simulink model "SIL_swarm_Vasarhelyi"  (R2020b)
settings: Solver=FixedStepAuto  StartTime=0.0  StopTime=T  FixedStep=sim_rate  RelTol=1e-3  EnableMultiTasking=on
model workspace (MAT data in the model file):
  SL_ROS_VariableLengthArrays_MaxSizes.CommonInfo.ArrayTruncateAction = 'EmitWarning'
  SL_ROS_VariableLengthArrays_MaxSizes.MsgTypeMap = containers.Map
  SL_ROS_VariableLengthArrays_MaxSizes.MsgTypeMap.serialization.keys = {'aircraft_communication/NetworkComm', 'aircraft_messages/Communication', 'aircraft_messages/NetworkComm'}
  SL_ROS_VariableLengthArrays_MaxSizes.MsgTypeMap.serialization.values{1}.PropertyName = 'Comms'
  SL_ROS_VariableLengthArrays_MaxSizes.MsgTypeMap.serialization.values{1}.DataType = 'aircraft_communication/Communication'
  SL_ROS_VariableLengthArrays_MaxSizes.MsgTypeMap.serialization.values{1}.MaxLength = 4
  SL_ROS_VariableLengthArrays_MaxSizes.MsgTypeMap.serialization.values{2}.PropertyName = 'Ssid'
  SL_ROS_VariableLengthArrays_MaxSizes.MsgTypeMap.serialization.values{2}.DataType = 'uint8'
  SL_ROS_VariableLengthArrays_MaxSizes.MsgTypeMap.serialization.values{2}.MaxLength = 8
  SL_ROS_VariableLengthArrays_MaxSizes.MsgTypeMap.serialization.values{3}.PropertyName = 'Comms'
  SL_ROS_VariableLengthArrays_MaxSizes.MsgTypeMap.serialization.values{3}.DataType = 'aircraft_messages/Communication'
  SL_ROS_VariableLengthArrays_MaxSizes.MsgTypeMap.serialization.values{3}.MaxLength = 8
  SL_ROS_VariableLengthArrays_MaxSizes.MsgTypeMap.serialization.uniformity = 0
  SL_ROS_VariableLengthArrays_MaxSizes.MsgTypeMap.serialization.keyType = 'char'
  SL_ROS_VariableLengthArrays_MaxSizes.MsgTypeMap.serialization.valueType = 'any'
undefined symbols (not defined in the file): airspeed_ref, Altitude_ref, DiscIntNeverNeededParam, Elevators, N_Waypoints, p_swarm, Propeller, Radius_waypoint, RightAileron, RightFlap, Rudder, Waypoints
libraries: robotlib x21, simulink x10, eeGeneralControl x5, dspvision x5
(part 1 of 4)
settings Model: Creator=fcsou  LastModifiedBy=fcsou
settings OptimizationCC: EnhancedBackFolding=on  PassReuseOutputArgsAs=Individual arguments  ZeroExternalMemoryAtStartup=off  ZeroInternalMemoryAtStartup=off  MaxStackSize=64  OptimizeBlockOrder=speed  DifferentSizesBufferReuse=on  OptimizationCustomize=off  EfficientTunableParamExpr=on
settings DebuggingCC: ParameterTunabilityLossMsg=error
settings HardwareCC: ProdBitPerPointer=32  ProdBitPerSizeT=32  ProdBitPerPtrDiffT=32  ProdLargestAtomicFloat=None  ProdIntDivRoundTo=Undefined  ProdEndianess=Unspecified  ProdWordSize=32  ProdHWDeviceType=Generic->Unspecified (assume 32-bit Generic)
settings ModelReferenceCC: PropagateSignalLabelsOutOfModel=off
settings SFSimCC: MATLABDynamicMemAlloc=off
settings RTWCC: Description=Embedded Coder  SystemTargetFile=ert.tlc  HardwareBoard=Robot Operating System (ROS)  TLCOptions="-aInlineSetEventsForThisBaseRateFcn=TLC_FALSE -aSuppressMultiTaskScheduler=TLC_FALSE  -aRateBasedStepFcn=0"  TemplateMakefile=ert_default_tmf  Toolchain=Catkin  TargetLang=C++
settings CodeAppCC: ForceParamTrailComments=on  IgnoreCustomStorageClasses=off  OperatorAnnotations=on  SimulinkDataObjDesc=on  SFDataObjDesc=on  InsertBlockDesc=on
settings ERTTargetCC: ERTCustomFileTemplate=rostime_codertarget_file_process.tlc

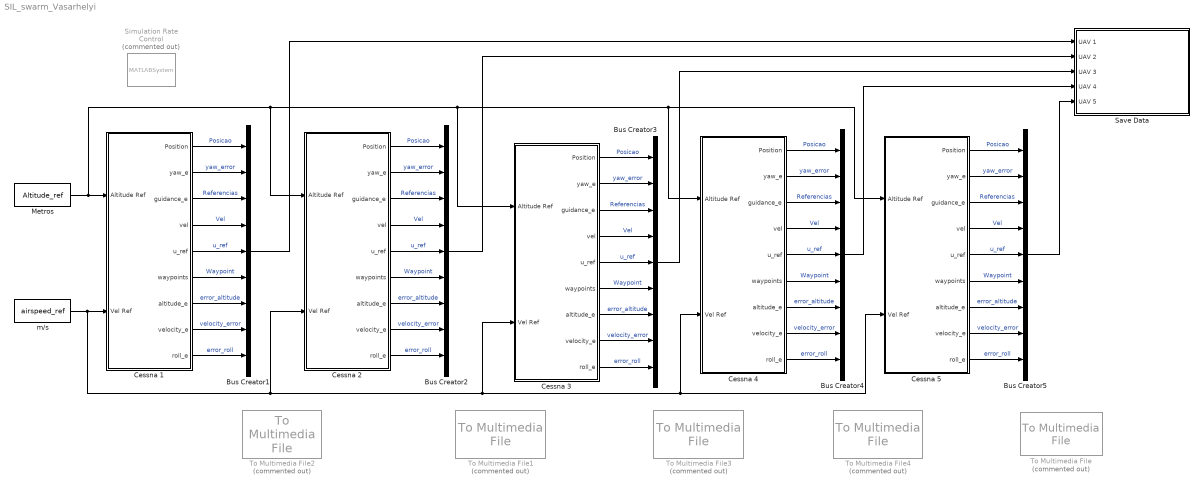
== system SIL_swarm_Vasarhelyi ==
  Bus Creator{1..5} (5 alike) : BusCreator  Inputs=9
  Cessna 1 : Subsystem
  Cessna 2 : Subsystem
  Cessna 3 : Subsystem
  Cessna 4 : Subsystem
  Cessna 5 : Subsystem
  Metros : Constant  Value=Altitude_ref
  Save Data : Subsystem
  Simulation Rate Control : MATLABSystem  Commented=on  System=ExampleHelperSimulationRateControl  SampleTime=0.01
      mask Type: ExampleHelperSimulationRateControl
      mask Display: disp('Rate Control');
  To Multimedia File : dspvision/To Multimedia File  Commented=on  outputFilename=C:\Tese\Results\results_swarm\uav5.mp4  streamSelection=Video only  videoCompressor=Lossy  audioCompressor=None (uncompressed)  imagePorts=One multidimensional signal  fileType=MPEG4  audioDatatype=Determine from input data type  fourcc=RGB  videoQuality=75  mj2000CompFactor=10
  To Multimedia File1 : dspvision/To Multimedia File  Commented=on  outputFilename=C:\Tese\Results\results_swarm\uav2.mp4  streamSelection=Video only  videoCompressor=None (uncompressed)  audioCompressor=None (uncompressed)  imagePorts=One multidimensional signal  fileType=MPEG4  audioDatatype=Determine from input data type  fourcc=RGB  videoQuality=75  mj2000CompFactor=10
  To Multimedia File2 : dspvision/To Multimedia File  Commented=on  outputFilename=C:\Tese\Results\results_swarm\uav1.mp4  streamSelection=Video only  videoCompressor=None (uncompressed)  audioCompressor=None (uncompressed)  imagePorts=One multidimensional signal  fileType=MPEG4  audioDatatype=Determine from input data type  fourcc=RGB  videoQuality=75  mj2000CompFactor=10
  To Multimedia File3 : dspvision/To Multimedia File  Commented=on  outputFilename=C:\Tese\Results\results_swarm\uav3.mp4  streamSelection=Video only  videoCompressor=None (uncompressed)  audioCompressor=None (uncompressed)  imagePorts=One multidimensional signal  fileType=MPEG4  audioDatatype=Determine from input data type  fourcc=RGB  videoQuality=75  mj2000CompFactor=10
  To Multimedia File4 : dspvision/To Multimedia File  Commented=on  outputFilename=C:\Tese\Results\results_swarm\uav4.mp4  streamSelection=Video only  videoCompressor=None (uncompressed)  audioCompressor=None (uncompressed)  imagePorts=One multidimensional signal  fileType=MPEG4  audioDatatype=Determine from input data type  fourcc=RGB  videoQuality=75  mj2000CompFactor=10
  m/s : Constant  Value=airspeed_ref
  wires:
  Bus Creator1/1 -> Save Data/1(UAV 1)
  Cessna 1/4(vel) -> Bus Creator1/4  "Vel"
  Cessna 1/5(u_ref) -> Bus Creator1/5  "u_ref"
  Cessna 1/1(Position) -> Bus Creator1/1  "Posicao"
  Cessna 1/2(yaw_e) -> Bus Creator1/2  "yaw_error"
  Cessna 1/8(velocity_e) -> Bus Creator1/8  "velocity_error"
  Cessna 1/7(altitude_e) -> Bus Creator1/7  "error_altitude"
  Cessna 1/6(waypoints) -> Bus Creator1/6  "Waypoint"
  Cessna 1/3(guidance_e) -> Bus Creator1/3  "Referencias"
  Cessna 1/9(roll_e) -> Bus Creator1/9  "error_roll"
  Cessna 2/9(roll_e) -> Bus Creator2/9  "error_roll"
  Cessna 2/3(guidance_e) -> Bus Creator2/3  "Referencias"
  Cessna 2/8(velocity_e) -> Bus Creator2/8  "velocity_error"
  Cessna 2/7(altitude_e) -> Bus Creator2/7  "error_altitude"
  Cessna 2/4(vel) -> Bus Creator2/4  "Vel"
  Cessna 2/6(waypoints) -> Bus Creator2/6  "Waypoint"
  Cessna 2/1(Position) -> Bus Creator2/1  "Posicao"
  Cessna 2/2(yaw_e) -> Bus Creator2/2  "yaw_error"
  Bus Creator2/1 -> Save Data/2(UAV 2)
  Cessna 2/5(u_ref) -> Bus Creator2/5  "u_ref"
  Cessna 3/9(roll_e) -> Bus Creator3/9  "error_roll"
  Cessna 3/3(guidance_e) -> Bus Creator3/3  "Referencias"
  Cessna 3/8(velocity_e) -> Bus Creator3/8  "velocity_error"
  Cessna 3/7(altitude_e) -> Bus Creator3/7  "error_altitude"
  Cessna 3/4(vel) -> Bus Creator3/4  "Vel"
  Cessna 3/6(waypoints) -> Bus Creator3/6  "Waypoint"
  Cessna 3/1(Position) -> Bus Creator3/1  "Posicao"
  Cessna 3/2(yaw_e) -> Bus Creator3/2  "yaw_error"
  Bus Creator3/1 -> Save Data/3(UAV 3)
  Cessna 3/5(u_ref) -> Bus Creator3/5  "u_ref"
  Cessna 4/9(roll_e) -> Bus Creator4/9  "error_roll"
  Cessna 4/3(guidance_e) -> Bus Creator4/3  "Referencias"
  Cessna 4/8(velocity_e) -> Bus Creator4/8  "velocity_error"
  Cessna 4/7(altitude_e) -> Bus Creator4/7  "error_altitude"
  Cessna 4/4(vel) -> Bus Creator4/4  "Vel"
  Cessna 4/6(waypoints) -> Bus Creator4/6  "Waypoint"
  Cessna 4/1(Position) -> Bus Creator4/1  "Posicao"
  Cessna 4/2(yaw_e) -> Bus Creator4/2  "yaw_error"
  Bus Creator4/1 -> Save Data/4(UAV 4)
  Cessna 4/5(u_ref) -> Bus Creator4/5  "u_ref"
  Metros/1 -> Cessna 4/1(Altitude Ref), Cessna 5/1(Altitude Ref), Cessna 3/1(Altitude Ref), Cessna 2/1(Altitude Ref), Cessna 1/1(Altitude Ref)
  Cessna 5/9(roll_e) -> Bus Creator5/9  "error_roll"
  Cessna 5/3(guidance_e) -> Bus Creator5/3  "Referencias"
  Cessna 5/8(velocity_e) -> Bus Creator5/8  "velocity_error"
  Cessna 5/7(altitude_e) -> Bus Creator5/7  "error_altitude"
  Cessna 5/4(vel) -> Bus Creator5/4  "Vel"
  Cessna 5/6(waypoints) -> Bus Creator5/6  "Waypoint"
  Cessna 5/1(Position) -> Bus Creator5/1  "Posicao"
  m/s/1 -> Cessna 5/2(Vel Ref), Cessna 4/2(Vel Ref), Cessna 3/2(Vel Ref), Cessna 2/2(Vel Ref), Cessna 1/2(Vel Ref)
  Cessna 5/2(yaw_e) -> Bus Creator5/2  "yaw_error"
  Bus Creator5/1 -> Save Data/5(UAV 5)
  Cessna 5/5(u_ref) -> Bus Creator5/5  "u_ref"

== system SIL_swarm_Vasarhelyi/Cessna 1 ==
  Altitude Ref : Inport
  Vel Ref : Inport  Port=2
  Attitude Control : Subsystem
      settings: PortSchema="{\"entries\":[{\"content\":{\"sides\":[{\"content\":{\"connectorIds\":[\"In1\",\"In2\",\"In3\",\"In4\",\"In5\",\"In6\"]},\"type\":\"ConnectorPlacement.EquallySpacedRectSide\",\"uuid\":\"f5987fb5-26bd-460f-ada3-c62a2cc917d9\"},{\"content\":{\"connectorIds\":[\"Out1\",\"Out2\",\"Out3\",\"Out4\"],\"side\":\"RIGHT\"},\"type\":\"ConnectorPlacement.EquallySpacedRectSide\",\"uuid\":\"78b4fbb6-b2d6-45e8-a79e-ccfb1aa742fa\"},{\"content\":{\"connectorIds\":[\"Out5\",\"Out6\",\"Out7\"],\"side\":\"TOP\"},\"type\":\"ConnectorPlacement.EquallySpacedRectSide\",\"uuid\":\"043ac8db-db42-42ba-ba46-d4f45f772f93\"},{\"content\":{\"connectorIds\":[],\"side\":\"HIDDEN\"},\"type\":\"ConnectorPlacement.EquallySpacedRectSide\",\"uuid\":\"557a5d68-6739-4613-818d-4b3751c4f08a\"}]},\"type\":\"ConnectorPlacement.EquallySpacedConnector\",\"uuid\":\"675ce67f-dd1b-4b16-8fb4-2c0be5e81414\"}],\"packageUris\":[\"http://schema.mathworks.com/mf0/Connector/R2020b\"],\"version\":\"1.0\"}"
  Bus Creator : BusCreator  Inputs=3
  Bus Creator1 : BusCreator  Inputs=3
  Bus Selector1 : BusSelector  OutputSignals=X,Y
  Controle de Direção : Subsystem
  High-Level : Subsystem
  ROS Communication : Subsystem
      settings: PortSchema="{\"entries\":[{\"content\":{\"sides\":[{\"content\":{\"connectorIds\":[\"In1\",\"In2\",\"In3\",\"In4\"]},\"type\":\"ConnectorPlacement.EquallySpacedRectSide\",\"uuid\":\"37ffebc2-6d57-4912-9ad0-de0bd75c512d\"},{\"content\":{\"connectorIds\":[\"Out1\",\"Out2\",\"Out3\",\"Out4\",\"Out5\",\"Out6\",\"Out7\"],\"side\":\"RIGHT\"},\"type\":\"ConnectorPlacement.EquallySpacedRectSide\",\"uuid\":\"870d0210-578f-4243-99d2-044c742eeea3\"},{\"content\":{\"connectorIds\":[\"Out8\"],\"side\":\"TOP\"},\"type\":\"ConnectorPlacement.EquallySpacedRectSide\",\"uuid\":\"d294e982-d3b3-4a84-8ae3-ca0953cabd4e\"},{\"content\":{\"connectorIds\":[],\"side\":\"HIDDEN\"},\"type\":\"ConnectorPlacement.EquallySpacedRectSide\",\"uuid\":\"f3838956-1f56-4acd-b9fa-f0f63fa39c9b\"}]},\"type\":\"ConnectorPlacement.EquallySpacedConnector\",\"uuid\":\"f2d40ee8-fbac-425c-83b3-c95127bc648e\"}],\"packageUris\":[\"http://schema.mathworks.com/mf0/Connector/R2020b\"],\"version\":\"1.0\"}"
  Position : Outport
  yaw_e : Outport  Port=2
  guidance_e : Outport  Port=3
  vel : Outport  Port=4
  u_ref : Outport  Port=5
  waypoints : Outport  Port=6
  altitude_e : Outport  Port=7
  velocity_e : Outport  Port=8
  roll_e : Outport  Port=9
  wires:
  Attitude Control/4(Throtlle) -> ROS Communication/4(Throttle)
  ROS Communication/2(Pitch) -> Bus Creator/2  "Pitch"
  Bus Selector1/2 -> Controle de Direção/3(Y)  "<Y>"
  Bus Selector1/1 -> Controle de Direção/2(X)  "<X>"
  Attitude Control/3(Aileron) -> ROS Communication/3(Aileron)
  ROS Communication/8(Xi) -> High-Level/3(Xi)
  Bus Creator/1 -> Attitude Control/2(Euler Angles)
  Attitude Control/2(Rudder) -> ROS Communication/2(Rudder)
  ROS Communication/5(ECEF X) -> Bus Creator1/2  "X"
  Controle de Direção/2(Roll Ref) -> Attitude Control/3(Roll_ref)
  Attitude Control/1(Profundor) -> ROS Communication/1(Profundor)
  Bus Creator1/1 -> Position/1, High-Level/1(Pos), Bus Selector1/1
  ROS Communication/6(ECEF Z) -> Attitude Control/4(Altitude), Bus Creator1/3  "Altitude"
  ROS Communication/7(Velocity) -> Attitude Control/5(Vel_in)
  Altitude Ref/1 -> Attitude Control/6(Altitude ref), High-Level/2(Altitude ref)
  High-Level/1(Y Ref) -> Controle de Direção/4(Y Ref)
  High-Level/2(X Ref) -> Controle de Direção/5(X Ref)
  ROS Communication/3(Yaw) -> Controle de Direção/1(Yaw), Bus Creator/3  "Yaw"
  ROS Communication/4(ECEF Y) -> Bus Creator1/1  "Y"
  ROS Communication/1(Roll) -> Bus Creator/1  "Roll"
  Controle de Direção/1(yaw_error) -> yaw_e/1
  Controle de Direção/3(guidance_error) -> guidance_e/1
  High-Level/3(vel) -> vel/1
  High-Level/4(u_ref) -> u_ref/1
  High-Level/5(Waypoints) -> waypoints/1
  Attitude Control/5(altitude_e) -> altitude_e/1
  Attitude Control/6(velocity_e) -> velocity_e/1
  Vel Ref/1 -> Attitude Control/1(Vel ref)
  Attitude Control/7(roll_e) -> roll_e/1

== system SIL_swarm_Vasarhelyi/Cessna 2 ==
  Altitude Ref : Inport
  Vel Ref : Inport  Port=2
  Attitude Control : Subsystem
      settings: PortSchema="{\"entries\":[{\"content\":{\"sides\":[{\"content\":{\"connectorIds\":[\"In1\",\"In2\",\"In3\",\"In4\",\"In5\",\"In6\"]},\"type\":\"ConnectorPlacement.EquallySpacedRectSide\",\"uuid\":\"f5987fb5-26bd-460f-ada3-c62a2cc917d9\"},{\"content\":{\"connectorIds\":[\"Out1\",\"Out2\",\"Out3\",\"Out4\"],\"side\":\"RIGHT\"},\"type\":\"ConnectorPlacement.EquallySpacedRectSide\",\"uuid\":\"78b4fbb6-b2d6-45e8-a79e-ccfb1aa742fa\"},{\"content\":{\"connectorIds\":[\"Out5\",\"Out6\",\"Out7\"],\"side\":\"TOP\"},\"type\":\"ConnectorPlacement.EquallySpacedRectSide\",\"uuid\":\"043ac8db-db42-42ba-ba46-d4f45f772f93\"},{\"content\":{\"connectorIds\":[],\"side\":\"HIDDEN\"},\"type\":\"ConnectorPlacement.EquallySpacedRectSide\",\"uuid\":\"557a5d68-6739-4613-818d-4b3751c4f08a\"}]},\"type\":\"ConnectorPlacement.EquallySpacedConnector\",\"uuid\":\"675ce67f-dd1b-4b16-8fb4-2c0be5e81414\"}],\"packageUris\":[\"http://schema.mathworks.com/mf0/Connector/R2020b\"],\"version\":\"1.0\"}"
  Bus Creator : BusCreator  Inputs=3
  Bus Creator1 : BusCreator  Inputs=3
  Bus Selector1 : BusSelector  OutputSignals=X,Y
  Controle de Direção : Subsystem
  High-Level : Subsystem
  ROS Communication : Subsystem
      settings: PortSchema="{\"entries\":[{\"content\":{\"sides\":[{\"content\":{\"connectorIds\":[\"In1\",\"In2\",\"In3\",\"In4\"]},\"type\":\"ConnectorPlacement.EquallySpacedRectSide\",\"uuid\":\"37ffebc2-6d57-4912-9ad0-de0bd75c512d\"},{\"content\":{\"connectorIds\":[\"Out1\",\"Out2\",\"Out3\",\"Out4\",\"Out5\",\"Out6\",\"Out7\"],\"side\":\"RIGHT\"},\"type\":\"ConnectorPlacement.EquallySpacedRectSide\",\"uuid\":\"870d0210-578f-4243-99d2-044c742eeea3\"},{\"content\":{\"connectorIds\":[\"Out8\"],\"side\":\"TOP\"},\"type\":\"ConnectorPlacement.EquallySpacedRectSide\",\"uuid\":\"d294e982-d3b3-4a84-8ae3-ca0953cabd4e\"},{\"content\":{\"connectorIds\":[],\"side\":\"HIDDEN\"},\"type\":\"ConnectorPlacement.EquallySpacedRectSide\",\"uuid\":\"f3838956-1f56-4acd-b9fa-f0f63fa39c9b\"}]},\"type\":\"ConnectorPlacement.EquallySpacedConnector\",\"uuid\":\"f2d40ee8-fbac-425c-83b3-c95127bc648e\"}],\"packageUris\":[\"http://schema.mathworks.com/mf0/Connector/R2020b\"],\"version\":\"1.0\"}"
  Position : Outport
  yaw_e : Outport  Port=2
  guidance_e : Outport  Port=3
  vel : Outport  Port=4
  u_ref : Outport  Port=5
  waypoints : Outport  Port=6
  altitude_e : Outport  Port=7
  velocity_e : Outport  Port=8
  roll_e : Outport  Port=9
  wires:
  Attitude Control/4(Throtlle) -> ROS Communication/4(Throttle)
  ROS Communication/2(Pitch) -> Bus Creator/2  "Pitch"
  Bus Selector1/2 -> Controle de Direção/3(Y)  "<Y>"
  Bus Selector1/1 -> Controle de Direção/2(X)  "<X>"
  Attitude Control/3(Aileron) -> ROS Communication/3(Aileron)
  ROS Communication/8(Xi) -> High-Level/3(Xi)
  Bus Creator/1 -> Attitude Control/2(Euler Angles)
  Attitude Control/2(Rudder) -> ROS Communication/2(Rudder)
  ROS Communication/5(ECEF X) -> Bus Creator1/2  "X"
  Controle de Direção/2(Roll Ref) -> Attitude Control/3(Roll_ref)
  Attitude Control/1(Profundor) -> ROS Communication/1(Profundor)
  Bus Creator1/1 -> Position/1, High-Level/1(Pos), Bus Selector1/1
  ROS Communication/6(ECEF Z) -> Attitude Control/4(Altitude), Bus Creator1/3  "Altitude"
  ROS Communication/7(Velocity) -> Attitude Control/5(Vel_in)
  Altitude Ref/1 -> Attitude Control/6(Altitude ref), High-Level/2(Altitude ref)
  High-Level/1(Y Ref) -> Controle de Direção/4(Y Ref)
  High-Level/2(X Ref) -> Controle de Direção/5(X Ref)
  ROS Communication/3(Yaw) -> Controle de Direção/1(Yaw), Bus Creator/3  "Yaw"
  ROS Communication/4(ECEF Y) -> Bus Creator1/1  "Y"
  ROS Communication/1(Roll) -> Bus Creator/1  "Roll"
  Controle de Direção/1(yaw_error) -> yaw_e/1
  Controle de Direção/3(guidance_error) -> guidance_e/1
  High-Level/3(vel) -> vel/1
  High-Level/4(u_ref) -> u_ref/1
  High-Level/5(Waypoints) -> waypoints/1
  Attitude Control/5(altitude_e) -> altitude_e/1
  Attitude Control/6(velocity_e) -> velocity_e/1
  Vel Ref/1 -> Attitude Control/1(Vel ref)
  Attitude Control/7(roll_e) -> roll_e/1

== system SIL_swarm_Vasarhelyi/Cessna 3 ==
  Altitude Ref : Inport
  Vel Ref : Inport  Port=2
  Attitude Control : Subsystem
      settings: PortSchema="{\"entries\":[{\"content\":{\"sides\":[{\"content\":{\"connectorIds\":[\"In1\",\"In2\",\"In3\",\"In4\",\"In5\",\"In6\"]},\"type\":\"ConnectorPlacement.EquallySpacedRectSide\",\"uuid\":\"f5987fb5-26bd-460f-ada3-c62a2cc917d9\"},{\"content\":{\"connectorIds\":[\"Out1\",\"Out2\",\"Out3\",\"Out4\"],\"side\":\"RIGHT\"},\"type\":\"ConnectorPlacement.EquallySpacedRectSide\",\"uuid\":\"78b4fbb6-b2d6-45e8-a79e-ccfb1aa742fa\"},{\"content\":{\"connectorIds\":[\"Out5\",\"Out6\",\"Out7\"],\"side\":\"TOP\"},\"type\":\"ConnectorPlacement.EquallySpacedRectSide\",\"uuid\":\"043ac8db-db42-42ba-ba46-d4f45f772f93\"},{\"content\":{\"connectorIds\":[],\"side\":\"HIDDEN\"},\"type\":\"ConnectorPlacement.EquallySpacedRectSide\",\"uuid\":\"557a5d68-6739-4613-818d-4b3751c4f08a\"}]},\"type\":\"ConnectorPlacement.EquallySpacedConnector\",\"uuid\":\"675ce67f-dd1b-4b16-8fb4-2c0be5e81414\"}],\"packageUris\":[\"http://schema.mathworks.com/mf0/Connector/R2020b\"],\"version\":\"1.0\"}"
  Bus Creator : BusCreator  Inputs=3
  Bus Creator1 : BusCreator  Inputs=3
  Bus Selector1 : BusSelector  OutputSignals=X,Y
  Controle de Direção : Subsystem
  High-Level : Subsystem
  ROS Communication : Subsystem
      settings: PortSchema="{\"entries\":[{\"content\":{\"sides\":[{\"content\":{\"connectorIds\":[\"In1\",\"In2\",\"In3\",\"In4\"]},\"type\":\"ConnectorPlacement.EquallySpacedRectSide\",\"uuid\":\"37ffebc2-6d57-4912-9ad0-de0bd75c512d\"},{\"content\":{\"connectorIds\":[\"Out1\",\"Out2\",\"Out3\",\"Out4\",\"Out5\",\"Out6\",\"Out7\"],\"side\":\"RIGHT\"},\"type\":\"ConnectorPlacement.EquallySpacedRectSide\",\"uuid\":\"870d0210-578f-4243-99d2-044c742eeea3\"},{\"content\":{\"connectorIds\":[\"Out8\"],\"side\":\"TOP\"},\"type\":\"ConnectorPlacement.EquallySpacedRectSide\",\"uuid\":\"d294e982-d3b3-4a84-8ae3-ca0953cabd4e\"},{\"content\":{\"connectorIds\":[],\"side\":\"HIDDEN\"},\"type\":\"ConnectorPlacement.EquallySpacedRectSide\",\"uuid\":\"f3838956-1f56-4acd-b9fa-f0f63fa39c9b\"}]},\"type\":\"ConnectorPlacement.EquallySpacedConnector\",\"uuid\":\"f2d40ee8-fbac-425c-83b3-c95127bc648e\"}],\"packageUris\":[\"http://schema.mathworks.com/mf0/Connector/R2020b\"],\"version\":\"1.0\"}"
  Position : Outport
  yaw_e : Outport  Port=2
  guidance_e : Outport  Port=3
  vel : Outport  Port=4
  u_ref : Outport  Port=5
  waypoints : Outport  Port=6
  altitude_e : Outport  Port=7
  velocity_e : Outport  Port=8
  roll_e : Outport  Port=9
  wires:
  Attitude Control/4(Throtlle) -> ROS Communication/4(Throttle)
  ROS Communication/2(Pitch) -> Bus Creator/2  "Pitch"
  Bus Selector1/2 -> Controle de Direção/3(Y)  "<Y>"
  Bus Selector1/1 -> Controle de Direção/2(X)  "<X>"
  Attitude Control/3(Aileron) -> ROS Communication/3(Aileron)
  ROS Communication/8(Xi) -> High-Level/3(Xi)
  Bus Creator/1 -> Attitude Control/2(Euler Angles)
  Attitude Control/2(Rudder) -> ROS Communication/2(Rudder)
  ROS Communication/5(ECEF X) -> Bus Creator1/2  "X"
  Controle de Direção/2(Roll Ref) -> Attitude Control/3(Roll_ref)
  Attitude Control/1(Profundor) -> ROS Communication/1(Profundor)
  Bus Creator1/1 -> Position/1, High-Level/1(Pos), Bus Selector1/1
  ROS Communication/6(ECEF Z) -> Attitude Control/4(Altitude), Bus Creator1/3  "Altitude"
  ROS Communication/7(Velocity) -> Attitude Control/5(Vel_in)
  Altitude Ref/1 -> Attitude Control/6(Altitude ref), High-Level/2(Altitude ref)
  High-Level/1(Y Ref) -> Controle de Direção/4(Y Ref)
  High-Level/2(X Ref) -> Controle de Direção/5(X Ref)
  ROS Communication/3(Yaw) -> Controle de Direção/1(Yaw), Bus Creator/3  "Yaw"
  ROS Communication/4(ECEF Y) -> Bus Creator1/1  "Y"
  ROS Communication/1(Roll) -> Bus Creator/1  "Roll"
  Controle de Direção/1(yaw_error) -> yaw_e/1
  Controle de Direção/3(guidance_error) -> guidance_e/1
  High-Level/3(vel) -> vel/1
  High-Level/4(u_ref) -> u_ref/1
  High-Level/5(Waypoints) -> waypoints/1
  Attitude Control/5(altitude_e) -> altitude_e/1
  Attitude Control/6(velocity_e) -> velocity_e/1
  Vel Ref/1 -> Attitude Control/1(Vel ref)
  Attitude Control/7(roll_e) -> roll_e/1

== system SIL_swarm_Vasarhelyi/Cessna 4 ==
  Altitude Ref : Inport
  Vel Ref : Inport  Port=2
  Attitude Control : Subsystem
      settings: PortSchema="{\"entries\":[{\"content\":{\"sides\":[{\"content\":{\"connectorIds\":[\"In1\",\"In2\",\"In3\",\"In4\",\"In5\",\"In6\"]},\"type\":\"ConnectorPlacement.EquallySpacedRectSide\",\"uuid\":\"f5987fb5-26bd-460f-ada3-c62a2cc917d9\"},{\"content\":{\"connectorIds\":[\"Out1\",\"Out2\",\"Out3\",\"Out4\"],\"side\":\"RIGHT\"},\"type\":\"ConnectorPlacement.EquallySpacedRectSide\",\"uuid\":\"78b4fbb6-b2d6-45e8-a79e-ccfb1aa742fa\"},{\"content\":{\"connectorIds\":[\"Out5\",\"Out6\",\"Out7\"],\"side\":\"TOP\"},\"type\":\"ConnectorPlacement.EquallySpacedRectSide\",\"uuid\":\"043ac8db-db42-42ba-ba46-d4f45f772f93\"},{\"content\":{\"connectorIds\":[],\"side\":\"HIDDEN\"},\"type\":\"ConnectorPlacement.EquallySpacedRectSide\",\"uuid\":\"557a5d68-6739-4613-818d-4b3751c4f08a\"}]},\"type\":\"ConnectorPlacement.EquallySpacedConnector\",\"uuid\":\"675ce67f-dd1b-4b16-8fb4-2c0be5e81414\"}],\"packageUris\":[\"http://schema.mathworks.com/mf0/Connector/R2020b\"],\"version\":\"1.0\"}"
  Bus Creator : BusCreator  Inputs=3
  Bus Creator1 : BusCreator  Inputs=3
  Bus Selector1 : BusSelector  OutputSignals=X,Y
  Controle de Direção : Subsystem
  High-Level : Subsystem
  ROS Communication : Subsystem
      settings: PortSchema="{\"entries\":[{\"content\":{\"sides\":[{\"content\":{\"connectorIds\":[\"In1\",\"In2\",\"In3\",\"In4\"]},\"type\":\"ConnectorPlacement.EquallySpacedRectSide\",\"uuid\":\"37ffebc2-6d57-4912-9ad0-de0bd75c512d\"},{\"content\":{\"connectorIds\":[\"Out1\",\"Out2\",\"Out3\",\"Out4\",\"Out5\",\"Out6\",\"Out7\"],\"side\":\"RIGHT\"},\"type\":\"ConnectorPlacement.EquallySpacedRectSide\",\"uuid\":\"870d0210-578f-4243-99d2-044c742eeea3\"},{\"content\":{\"connectorIds\":[\"Out8\"],\"side\":\"TOP\"},\"type\":\"ConnectorPlacement.EquallySpacedRectSide\",\"uuid\":\"d294e982-d3b3-4a84-8ae3-ca0953cabd4e\"},{\"content\":{\"connectorIds\":[],\"side\":\"HIDDEN\"},\"type\":\"ConnectorPlacement.EquallySpacedRectSide\",\"uuid\":\"f3838956-1f56-4acd-b9fa-f0f63fa39c9b\"}]},\"type\":\"ConnectorPlacement.EquallySpacedConnector\",\"uuid\":\"f2d40ee8-fbac-425c-83b3-c95127bc648e\"}],\"packageUris\":[\"http://schema.mathworks.com/mf0/Connector/R2020b\"],\"version\":\"1.0\"}"
  Position : Outport
  yaw_e : Outport  Port=2
  guidance_e : Outport  Port=3
  vel : Outport  Port=4
  u_ref : Outport  Port=5
  waypoints : Outport  Port=6
  altitude_e : Outport  Port=7
  velocity_e : Outport  Port=8
  roll_e : Outport  Port=9
  wires:
  Attitude Control/4(Throtlle) -> ROS Communication/4(Throttle)
  ROS Communication/2(Pitch) -> Bus Creator/2  "Pitch"
  Bus Selector1/2 -> Controle de Direção/3(Y)  "<Y>"
  Bus Selector1/1 -> Controle de Direção/2(X)  "<X>"
  Attitude Control/3(Aileron) -> ROS Communication/3(Aileron)
  ROS Communication/8(Xi) -> High-Level/3(Xi)
  Bus Creator/1 -> Attitude Control/2(Euler Angles)
  Attitude Control/2(Rudder) -> ROS Communication/2(Rudder)
  ROS Communication/5(ECEF X) -> Bus Creator1/2  "X"
  Controle de Direção/2(Roll Ref) -> Attitude Control/3(Roll_ref)
  Attitude Control/1(Profundor) -> ROS Communication/1(Profundor)
  Bus Creator1/1 -> Position/1, High-Level/1(Pos), Bus Selector1/1
  ROS Communication/6(ECEF Z) -> Attitude Control/4(Altitude), Bus Creator1/3  "Altitude"
  ROS Communication/7(Velocity) -> Attitude Control/5(Vel_in)
  Altitude Ref/1 -> Attitude Control/6(Altitude ref), High-Level/2(Altitude ref)
  High-Level/1(Y Ref) -> Controle de Direção/4(Y Ref)
  High-Level/2(X Ref) -> Controle de Direção/5(X Ref)
  ROS Communication/3(Yaw) -> Controle de Direção/1(Yaw), Bus Creator/3  "Yaw"
  ROS Communication/4(ECEF Y) -> Bus Creator1/1  "Y"
  ROS Communication/1(Roll) -> Bus Creator/1  "Roll"
  Controle de Direção/1(yaw_error) -> yaw_e/1
  Controle de Direção/3(guidance_error) -> guidance_e/1
  High-Level/3(vel) -> vel/1
  High-Level/4(u_ref) -> u_ref/1
  High-Level/5(Waypoints) -> waypoints/1
  Attitude Control/5(altitude_e) -> altitude_e/1
  Attitude Control/6(velocity_e) -> velocity_e/1
  Vel Ref/1 -> Attitude Control/1(Vel ref)
  Attitude Control/7(roll_e) -> roll_e/1

== system SIL_swarm_Vasarhelyi/Cessna 5 ==
  Altitude Ref : Inport
  Vel Ref : Inport  Port=2
  Attitude Control : Subsystem
      settings: PortSchema="{\"entries\":[{\"content\":{\"sides\":[{\"content\":{\"connectorIds\":[\"In1\",\"In2\",\"In3\",\"In4\",\"In5\",\"In6\"]},\"type\":\"ConnectorPlacement.EquallySpacedRectSide\",\"uuid\":\"f5987fb5-26bd-460f-ada3-c62a2cc917d9\"},{\"content\":{\"connectorIds\":[\"Out1\",\"Out2\",\"Out3\",\"Out4\"],\"side\":\"RIGHT\"},\"type\":\"ConnectorPlacement.EquallySpacedRectSide\",\"uuid\":\"78b4fbb6-b2d6-45e8-a79e-ccfb1aa742fa\"},{\"content\":{\"connectorIds\":[\"Out5\",\"Out6\",\"Out7\"],\"side\":\"TOP\"},\"type\":\"ConnectorPlacement.EquallySpacedRectSide\",\"uuid\":\"043ac8db-db42-42ba-ba46-d4f45f772f93\"},{\"content\":{\"connectorIds\":[],\"side\":\"HIDDEN\"},\"type\":\"ConnectorPlacement.EquallySpacedRectSide\",\"uuid\":\"557a5d68-6739-4613-818d-4b3751c4f08a\"}]},\"type\":\"ConnectorPlacement.EquallySpacedConnector\",\"uuid\":\"675ce67f-dd1b-4b16-8fb4-2c0be5e81414\"}],\"packageUris\":[\"http://schema.mathworks.com/mf0/Connector/R2020b\"],\"version\":\"1.0\"}"
  Bus Creator : BusCreator  Inputs=3
  Bus Creator1 : BusCreator  Inputs=3
  Bus Selector1 : BusSelector  OutputSignals=X,Y
  Controle de Direção : Subsystem
  High-Level : Subsystem
  ROS Communication : Subsystem
      settings: PortSchema="{\"entries\":[{\"content\":{\"sides\":[{\"content\":{\"connectorIds\":[\"In1\",\"In2\",\"In3\",\"In4\"]},\"type\":\"ConnectorPlacement.EquallySpacedRectSide\",\"uuid\":\"37ffebc2-6d57-4912-9ad0-de0bd75c512d\"},{\"content\":{\"connectorIds\":[\"Out1\",\"Out2\",\"Out3\",\"Out4\",\"Out5\",\"Out6\",\"Out7\"],\"side\":\"RIGHT\"},\"type\":\"ConnectorPlacement.EquallySpacedRectSide\",\"uuid\":\"870d0210-578f-4243-99d2-044c742eeea3\"},{\"content\":{\"connectorIds\":[\"Out8\"],\"side\":\"TOP\"},\"type\":\"ConnectorPlacement.EquallySpacedRectSide\",\"uuid\":\"d294e982-d3b3-4a84-8ae3-ca0953cabd4e\"},{\"content\":{\"connectorIds\":[],\"side\":\"HIDDEN\"},\"type\":\"ConnectorPlacement.EquallySpacedRectSide\",\"uuid\":\"f3838956-1f56-4acd-b9fa-f0f63fa39c9b\"}]},\"type\":\"ConnectorPlacement.EquallySpacedConnector\",\"uuid\":\"f2d40ee8-fbac-425c-83b3-c95127bc648e\"}],\"packageUris\":[\"http://schema.mathworks.com/mf0/Connector/R2020b\"],\"version\":\"1.0\"}"
  Position : Outport
  yaw_e : Outport  Port=2
  guidance_e : Outport  Port=3
  vel : Outport  Port=4
  u_ref : Outport  Port=5
  waypoints : Outport  Port=6
  altitude_e : Outport  Port=7
  velocity_e : Outport  Port=8
  roll_e : Outport  Port=9
  wires:
  Attitude Control/4(Throtlle) -> ROS Communication/4(Throttle)
  ROS Communication/2(Pitch) -> Bus Creator/2  "Pitch"
  Bus Selector1/2 -> Controle de Direção/3(Y)  "<Y>"
  Bus Selector1/1 -> Controle de Direção/2(X)  "<X>"
  Attitude Control/3(Aileron) -> ROS Communication/3(Aileron)
  ROS Communication/8(Xi) -> High-Level/3(Xi)
  Bus Creator/1 -> Attitude Control/2(Euler Angles)
  Attitude Control/2(Rudder) -> ROS Communication/2(Rudder)
  ROS Communication/5(ECEF X) -> Bus Creator1/2  "X"
  Controle de Direção/2(Roll Ref) -> Attitude Control/3(Roll_ref)
  Attitude Control/1(Profundor) -> ROS Communication/1(Profundor)
  Bus Creator1/1 -> Position/1, High-Level/1(Pos), Bus Selector1/1
  ROS Communication/6(ECEF Z) -> Attitude Control/4(Altitude), Bus Creator1/3  "Altitude"
  ROS Communication/7(Velocity) -> Attitude Control/5(Vel_in)
  Altitude Ref/1 -> Attitude Control/6(Altitude ref), High-Level/2(Altitude ref)
  High-Level/1(Y Ref) -> Controle de Direção/4(Y Ref)
  High-Level/2(X Ref) -> Controle de Direção/5(X Ref)
  ROS Communication/3(Yaw) -> Controle de Direção/1(Yaw), Bus Creator/3  "Yaw"
  ROS Communication/4(ECEF Y) -> Bus Creator1/1  "Y"
  ROS Communication/1(Roll) -> Bus Creator/1  "Roll"
  Controle de Direção/1(yaw_error) -> yaw_e/1
  Controle de Direção/3(guidance_error) -> guidance_e/1
  High-Level/3(vel) -> vel/1
  High-Level/4(u_ref) -> u_ref/1
  High-Level/5(Waypoints) -> waypoints/1
  Attitude Control/5(altitude_e) -> altitude_e/1
  Attitude Control/6(velocity_e) -> velocity_e/1
  Vel Ref/1 -> Attitude Control/1(Vel ref)
  Attitude Control/7(roll_e) -> roll_e/1

== system SIL_swarm_Vasarhelyi/Save Data ==
  UAV 1 : Inport
  UAV 2 : Inport  Port=2
  UAV 3 : Inport  Port=3
  UAV 4 : Inport  Port=4
  UAV 5 : Inport  Port=5
  Current Time : robotlib/Current Time  OutputFormat=double  SampleTime=-1  ModelName=SIL_swarm_Vasarhelyi
      settings: SourceProductBaseCode=RR
  To Workspace1 : ToWorkspace  VariableName=UAV1  SaveFormat=Timeseries  SampleTime=-1
  To Workspace2 : ToWorkspace  VariableName=UAV2  SaveFormat=Timeseries  SampleTime=-1
  To Workspace3 : ToWorkspace  VariableName=UAV3  SaveFormat=Timeseries  SampleTime=-1
  To Workspace4 : ToWorkspace  VariableName=UAV4  SaveFormat=Timeseries  SampleTime=-1
  To Workspace5 : ToWorkspace  VariableName=UAV5  SaveFormat=Timeseries  SampleTime=-1
  To Workspace6 : ToWorkspace  VariableName=ROStime  SaveFormat=Timeseries  SampleTime=-1
  wires:
  UAV 1/1 -> To Workspace1/1
  UAV 2/1 -> To Workspace2/1
  UAV 3/1 -> To Workspace3/1
  UAV 4/1 -> To Workspace4/1
  UAV 5/1 -> To Workspace5/1
  Current Time/1 -> To Workspace6/1

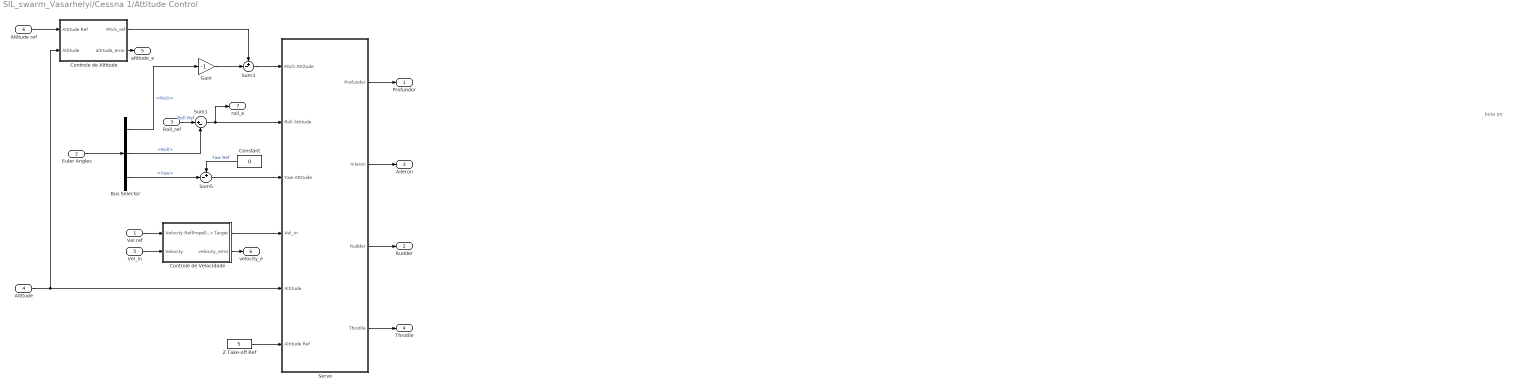
== system SIL_swarm_Vasarhelyi/Cessna 1/Attitude Control ==
  note: bota po
  Vel ref : Inport
  Euler Angles : Inport  Port=2
  Roll_ref : Inport  Port=3
  Altitude : Inport  Port=4
  Vel_in : Inport  Port=5
  Altitude ref : Inport  Port=6
  Bus Selector : BusSelector  OutputSignals=Pitch,Roll,Yaw
  Constant : Constant  Value=0
  Controle de Altitude : Subsystem
  Controle de Velocidade : Subsystem
  Gain : Gain  Gain=-1
  Servo : Subsystem
  Sum1 : Sum  Inputs=|+-
  Sum3 : Sum  Inputs=+-|
  Sum5 : Sum  Inputs=+-|
  Z Take-off Ref : Constant  Value=5
  Profundor : Outport
  Rudder : Outport  Port=2
  Aileron : Outport  Port=3
  Throtlle : Outport  Port=4
  altitude_e : Outport  Port=5
  velocity_e : Outport  Port=6
  roll_e : Outport  Port=7
  wires:
  Roll_ref/1 -> Sum1/1  "Roll Ref"
  Constant/1 -> Sum5/1  "Yaw Ref"
  Servo/4(Throtlle) -> Throtlle/1
  Servo/2(Aileron) -> Aileron/1
  Servo/3(Rudder) -> Rudder/1
  Servo/1(Profundor) -> Profundor/1
  Z Take-off Ref/1 -> Servo/6(Altitude Ref)
  Altitude/1 -> Controle de Altitude/2(Altitude), Servo/5(Altitude)
  Gain/1 -> Sum3/2
  Sum5/1 -> Servo/3(Yaw Attitude)
  Bus Selector/3 -> Sum5/2  "<Yaw>"
  Sum3/1 -> Servo/1(Pitch Attitude)
  Euler Angles/1 -> Bus Selector/1
  Bus Selector/1 -> Gain/1  "<Pitch>"
  Bus Selector/2 -> Sum1/2  "<Roll>"
  Controle de Velocidade/1(Propeller Target) -> Servo/4(Vel_in)
  Controle de Altitude/1(Pitch_ref) -> Sum3/1
  Vel ref/1 -> Controle de Velocidade/1(Velocity Ref)
  Altitude ref/1 -> Controle de Altitude/1(Altitude Ref)
  Sum1/1 -> roll_e/1, Servo/2(Roll Attitude)
  Vel_in/1 -> Controle de Velocidade/2(Velocity)
  Controle de Altitude/2(altitude_error) -> altitude_e/1
  Controle de Velocidade/2(velocity_error) -> velocity_e/1

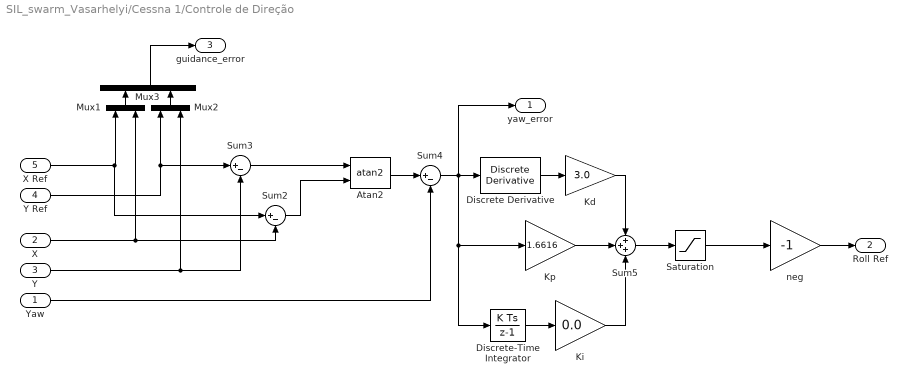
== system SIL_swarm_Vasarhelyi/Cessna 1/Controle de Direção ==
  Yaw : Inport
  X : Inport  Port=2
  Y : Inport  Port=3
  Y Ref : Inport  Port=4
  X Ref : Inport  Port=5
  Atan2 : Trigonometry  Operator=atan2
  Discrete Derivative : simulink/Discrete/Discrete Derivative  gainval=1.0  ICPrevScaledInput=0.0  OutMin=[]  OutMax=[]  OutDataType=fixdt(1, 16)  OutScaling=2^-10  DoSatur=off
  Discrete-Time Integrator : DiscreteIntegrator  SampleTime=-1  ICPrevOutput=DiscIntNeverNeededParam  ICPrevScaledInput=DiscIntNeverNeededParam
  Kd : Gain  Gain=3.0
  Ki : Gain  Gain=0.0
  Kp : Gain  Gain=1.6616
  Mux1 : Mux  Inputs=2
  Mux2 : Mux  Inputs=2
  Mux3 : Mux  Inputs=2
  Saturation : Saturate  UpperLimit=0.226893  LowerLimit=-0.226893
  Sum2 : Sum  Inputs=|+-
  Sum3 : Sum  Inputs=|+-
  Sum4 : Sum  Inputs=|+-
  Sum5 : Sum  Inputs=+++
  neg : Gain  Gain=-1
  yaw_error : Outport
  Roll Ref : Outport  Port=2
  guidance_error : Outport  Port=3
  wires:
  Mux1/1 -> Mux3/1
  Mux2/1 -> Mux3/2
  Saturation/1 -> neg/1
  neg/1 -> Roll Ref/1
  Sum3/1 -> Atan2/1
  Y/1 -> Sum3/2, Mux2/2
  Y Ref/1 -> Sum3/1, Mux2/1
  X Ref/1 -> Sum2/1, Mux1/1
  X/1 -> Sum2/2, Mux1/2
  Sum2/1 -> Atan2/2
  Atan2/1 -> Sum4/1
  Yaw/1 -> Sum4/2
  Mux3/1 -> guidance_error/1
  Sum5/1 -> Saturation/1
  Kp/1 -> Sum5/2
  Kd/1 -> Sum5/1
  Discrete Derivative/1 -> Kd/1
  Discrete-Time Integrator/1 -> Ki/1
  Sum4/1 -> Discrete-Time Integrator/1, Kp/1, Discrete Derivative/1, yaw_error/1
  Ki/1 -> Sum5/3

== system SIL_swarm_Vasarhelyi/Cessna 1/High-Level ==
  Pos : Inport
  Altitude ref : Inport  Port=2
  Xi : Inport  Port=3
  Bus Selector2 : BusSelector  OutputSignals=X,Y,Altitude
  Filtered Derivative Discrete : eeGeneralControl/Filtered Derivative (Discrete or Continuous)  K=1  T=0.001  B=inf  A=-inf  minRatio=10  init_option=Inherited from block input  x0=0  Ts=-1
      settings: SourceProductBaseCode=PS
  Gerador de Waypoints : Subsystem
  Mux : Mux  Inputs=3
  Mux1 : Mux  Inputs=3
  Terminator2 : Terminator
  Vasarhelyi Algorithm : Subsystem
  Velocity Direction : MATLAB Function  TreatAsAtomicUnit=on
  Y Ref : Outport
  X Ref : Outport  Port=2
  vel : Outport  Port=3
  u_ref : Outport  Port=4
  Waypoints : Outport  Port=5
  wires:
  Mux1/1 -> Waypoints/1, Velocity Direction/2(wp)
  Velocity Direction/1(u_ref) -> u_ref/1, Vasarhelyi Algorithm/3(u_ref)
  Pos/1 -> Bus Selector2/1
  Altitude ref/1 -> Mux1/3
  Gerador de Waypoints/2(Y Ref) -> Mux1/2
  Gerador de Waypoints/1(X Ref) -> Mux1/1
  Bus Selector2/1 -> Mux/1  "<X>"
  Bus Selector2/2 -> Mux/2  "<Y>"
  Bus Selector2/3 -> Mux/3  "<Altitude>"
  Mux/1 -> Filtered Derivative Discrete/1, Vasarhelyi Algorithm/1(pos_i), Velocity Direction/1(pos)
  Filtered Derivative Discrete/1 -> vel/1
  Xi/1 -> Vasarhelyi Algorithm/2(pqj)
  Vasarhelyi Algorithm/1(X) -> X Ref/1
  Vasarhelyi Algorithm/2(Y) -> Y Ref/1
  Vasarhelyi Algorithm/3(Z) -> Terminator2/1
  Vasarhelyi Algorithm/4(Xi) -> Gerador de Waypoints/1(Xi)

== system SIL_swarm_Vasarhelyi/Cessna 1/ROS Communication ==
  Profundor : Inport
  Rudder : Inport  Port=2
  Aileron : Inport  Port=3
  Throttle : Inport  Port=4
  Constant : Constant  Value=0
  Constant1 : Constant  Value=0
  Envio e Recepção de Dados do ROS : Subsystem
  Terminator2 : Terminator
  Roll : Outport
  Pitch : Outport  Port=2
  Yaw : Outport  Port=3
  ECEF Y : Outport  Port=4
  ECEF X : Outport  Port=5
  ECEF Z : Outport  Port=6
  Velocity : Outport  Port=7
  Xi : Outport  Port=8
  wires:
  Profundor/1 -> Envio e Recepção de Dados do ROS/2(Elevators)
  Constant/1 -> Envio e Recepção de Dados do ROS/3(Flap)
  Aileron/1 -> Envio e Recepção de Dados do ROS/4(Aileron)
  Envio e Recepção de Dados do ROS/1(Pitch) -> Pitch/1
  Envio e Recepção de Dados do ROS/4(ECEF X) -> ECEF X/1
  Envio e Recepção de Dados do ROS/5(ECEF Y) -> ECEF Y/1
  Envio e Recepção de Dados do ROS/2(Yaw) -> Yaw/1
  Envio e Recepção de Dados do ROS/3(Roll) -> Roll/1
  Envio e Recepção de Dados do ROS/6(ECEF Z) -> ECEF Z/1
  Envio e Recepção de Dados do ROS/7(Velocity) -> Velocity/1
  Rudder/1 -> Terminator2/1
  Envio e Recepção de Dados do ROS/8(Xi) -> Xi/1
  Throttle/1 -> Envio e Recepção de Dados do ROS/5(Propeller)
  Constant1/1 -> Envio e Recepção de Dados do ROS/1(Rudder)

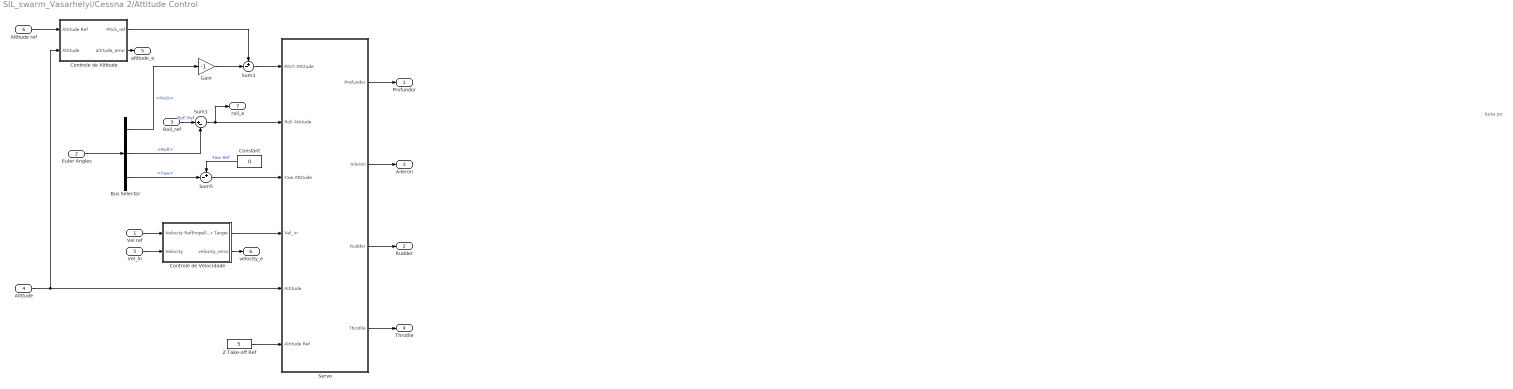
== system SIL_swarm_Vasarhelyi/Cessna 2/Attitude Control ==
  note: bota po
  Vel ref : Inport
  Euler Angles : Inport  Port=2
  Roll_ref : Inport  Port=3
  Altitude : Inport  Port=4
  Vel_in : Inport  Port=5
  Altitude ref : Inport  Port=6
  Bus Selector : BusSelector  OutputSignals=Pitch,Roll,Yaw
  Constant : Constant  Value=0
  Controle de Altitude : Subsystem
  Controle de Velocidade : Subsystem
  Gain : Gain  Gain=-1
  Servo : Subsystem
  Sum1 : Sum  Inputs=|+-
  Sum3 : Sum  Inputs=+-|
  Sum5 : Sum  Inputs=+-|
  Z Take-off Ref : Constant  Value=5
  Profundor : Outport
  Rudder : Outport  Port=2
  Aileron : Outport  Port=3
  Throtlle : Outport  Port=4
  altitude_e : Outport  Port=5
  velocity_e : Outport  Port=6
  roll_e : Outport  Port=7
  wires:
  Roll_ref/1 -> Sum1/1  "Roll Ref"
  Constant/1 -> Sum5/1  "Yaw Ref"
  Servo/4(Throtlle) -> Throtlle/1
  Servo/2(Aileron) -> Aileron/1
  Servo/3(Rudder) -> Rudder/1
  Servo/1(Profundor) -> Profundor/1
  Z Take-off Ref/1 -> Servo/6(Altitude Ref)
  Altitude/1 -> Controle de Altitude/2(Altitude), Servo/5(Altitude)
  Gain/1 -> Sum3/2
  Sum5/1 -> Servo/3(Yaw Attitude)
  Bus Selector/3 -> Sum5/2  "<Yaw>"
  Sum3/1 -> Servo/1(Pitch Attitude)
  Euler Angles/1 -> Bus Selector/1
  Bus Selector/1 -> Gain/1  "<Pitch>"
  Bus Selector/2 -> Sum1/2  "<Roll>"
  Controle de Velocidade/1(Propeller Target) -> Servo/4(Vel_in)
  Controle de Altitude/1(Pitch_ref) -> Sum3/1
  Vel ref/1 -> Controle de Velocidade/1(Velocity Ref)
  Altitude ref/1 -> Controle de Altitude/1(Altitude Ref)
  Sum1/1 -> roll_e/1, Servo/2(Roll Attitude)
  Vel_in/1 -> Controle de Velocidade/2(Velocity)
  Controle de Altitude/2(altitude_error) -> altitude_e/1
  Controle de Velocidade/2(velocity_error) -> velocity_e/1

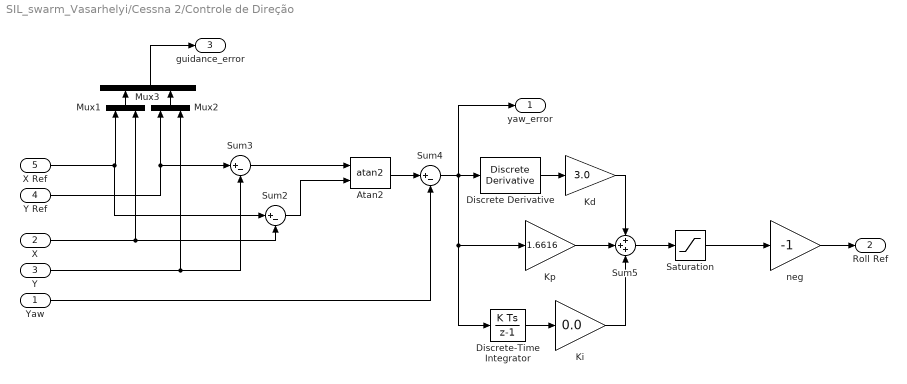
== system SIL_swarm_Vasarhelyi/Cessna 2/Controle de Direção ==
  Yaw : Inport
  X : Inport  Port=2
  Y : Inport  Port=3
  Y Ref : Inport  Port=4
  X Ref : Inport  Port=5
  Atan2 : Trigonometry  Operator=atan2
  Discrete Derivative : simulink/Discrete/Discrete Derivative  gainval=1.0  ICPrevScaledInput=0.0  OutMin=[]  OutMax=[]  OutDataType=fixdt(1, 16)  OutScaling=2^-10  DoSatur=off
  Discrete-Time Integrator : DiscreteIntegrator  SampleTime=-1  ICPrevOutput=DiscIntNeverNeededParam  ICPrevScaledInput=DiscIntNeverNeededParam
  Kd : Gain  Gain=3.0
  Ki : Gain  Gain=0.0
  Kp : Gain  Gain=1.6616
  Mux1 : Mux  Inputs=2
  Mux2 : Mux  Inputs=2
  Mux3 : Mux  Inputs=2
  Saturation : Saturate  UpperLimit=0.226893  LowerLimit=-0.226893
  Sum2 : Sum  Inputs=|+-
  Sum3 : Sum  Inputs=|+-
  Sum4 : Sum  Inputs=|+-
  Sum5 : Sum  Inputs=+++
  neg : Gain  Gain=-1
  yaw_error : Outport
  Roll Ref : Outport  Port=2
  guidance_error : Outport  Port=3
  wires:
  Mux1/1 -> Mux3/1
  Mux2/1 -> Mux3/2
  Saturation/1 -> neg/1
  neg/1 -> Roll Ref/1
  Sum3/1 -> Atan2/1
  Y/1 -> Sum3/2, Mux2/2
  Y Ref/1 -> Sum3/1, Mux2/1
  X Ref/1 -> Sum2/1, Mux1/1
  X/1 -> Sum2/2, Mux1/2
  Sum2/1 -> Atan2/2
  Atan2/1 -> Sum4/1
  Yaw/1 -> Sum4/2
  Mux3/1 -> guidance_error/1
  Sum5/1 -> Saturation/1
  Kp/1 -> Sum5/2
  Kd/1 -> Sum5/1
  Discrete Derivative/1 -> Kd/1
  Discrete-Time Integrator/1 -> Ki/1
  Sum4/1 -> Discrete-Time Integrator/1, Kp/1, Discrete Derivative/1, yaw_error/1
  Ki/1 -> Sum5/3

== system SIL_swarm_Vasarhelyi/Cessna 2/High-Level ==
  Pos : Inport
  Altitude ref : Inport  Port=2
  Xi : Inport  Port=3
  Bus Selector2 : BusSelector  OutputSignals=X,Y,Altitude
  Filtered Derivative Discrete : eeGeneralControl/Filtered Derivative (Discrete or Continuous)  K=1  T=0.001  B=inf  A=-inf  minRatio=10  init_option=Inherited from block input  x0=0  Ts=-1
      settings: SourceProductBaseCode=PS
  Gerador de Waypoints : Subsystem
  Mux : Mux  Inputs=3
  Mux1 : Mux  Inputs=3
  Terminator2 : Terminator
  Vasarhelyi Algorithm : Subsystem
  Velocity Direction : MATLAB Function  TreatAsAtomicUnit=on
  Y Ref : Outport
  X Ref : Outport  Port=2
  vel : Outport  Port=3
  u_ref : Outport  Port=4
  Waypoints : Outport  Port=5
  wires:
  Mux1/1 -> Waypoints/1, Velocity Direction/2(wp)
  Velocity Direction/1(u_ref) -> u_ref/1, Vasarhelyi Algorithm/3(u_ref)
  Pos/1 -> Bus Selector2/1
  Altitude ref/1 -> Mux1/3
  Gerador de Waypoints/2(Y Ref) -> Mux1/2
  Gerador de Waypoints/1(X Ref) -> Mux1/1
  Bus Selector2/1 -> Mux/1  "<X>"
  Bus Selector2/2 -> Mux/2  "<Y>"
  Bus Selector2/3 -> Mux/3  "<Altitude>"
  Mux/1 -> Filtered Derivative Discrete/1, Vasarhelyi Algorithm/1(pos_i), Velocity Direction/1(pos)
  Filtered Derivative Discrete/1 -> vel/1
  Xi/1 -> Vasarhelyi Algorithm/2(pqj)
  Vasarhelyi Algorithm/1(X) -> X Ref/1
  Vasarhelyi Algorithm/2(Y) -> Y Ref/1
  Vasarhelyi Algorithm/3(Z) -> Terminator2/1
  Vasarhelyi Algorithm/4(Xi) -> Gerador de Waypoints/1(Xi)

== system SIL_swarm_Vasarhelyi/Cessna 2/ROS Communication ==
  Profundor : Inport
  Rudder : Inport  Port=2
  Aileron : Inport  Port=3
  Throttle : Inport  Port=4
  Constant : Constant  Value=0
  Constant1 : Constant  Value=0
  Envio e Recepção de Dados do ROS : Subsystem
  Terminator2 : Terminator
  Roll : Outport
  Pitch : Outport  Port=2
  Yaw : Outport  Port=3
  ECEF Y : Outport  Port=4
  ECEF X : Outport  Port=5
  ECEF Z : Outport  Port=6
  Velocity : Outport  Port=7
  Xi : Outport  Port=8
  wires:
  Profundor/1 -> Envio e Recepção de Dados do ROS/2(Elevators)
  Constant/1 -> Envio e Recepção de Dados do ROS/3(Flap)
  Aileron/1 -> Envio e Recepção de Dados do ROS/4(Aileron)
  Envio e Recepção de Dados do ROS/1(Pitch) -> Pitch/1
  Envio e Recepção de Dados do ROS/4(ECEF X) -> ECEF X/1
  Envio e Recepção de Dados do ROS/5(ECEF Y) -> ECEF Y/1
  Envio e Recepção de Dados do ROS/2(Yaw) -> Yaw/1
  Envio e Recepção de Dados do ROS/3(Roll) -> Roll/1
  Envio e Recepção de Dados do ROS/6(ECEF Z) -> ECEF Z/1
  Envio e Recepção de Dados do ROS/7(Velocity) -> Velocity/1
  Rudder/1 -> Terminator2/1
  Envio e Recepção de Dados do ROS/8(Xi) -> Xi/1
  Throttle/1 -> Envio e Recepção de Dados do ROS/5(Propeller)
  Constant1/1 -> Envio e Recepção de Dados do ROS/1(Rudder)

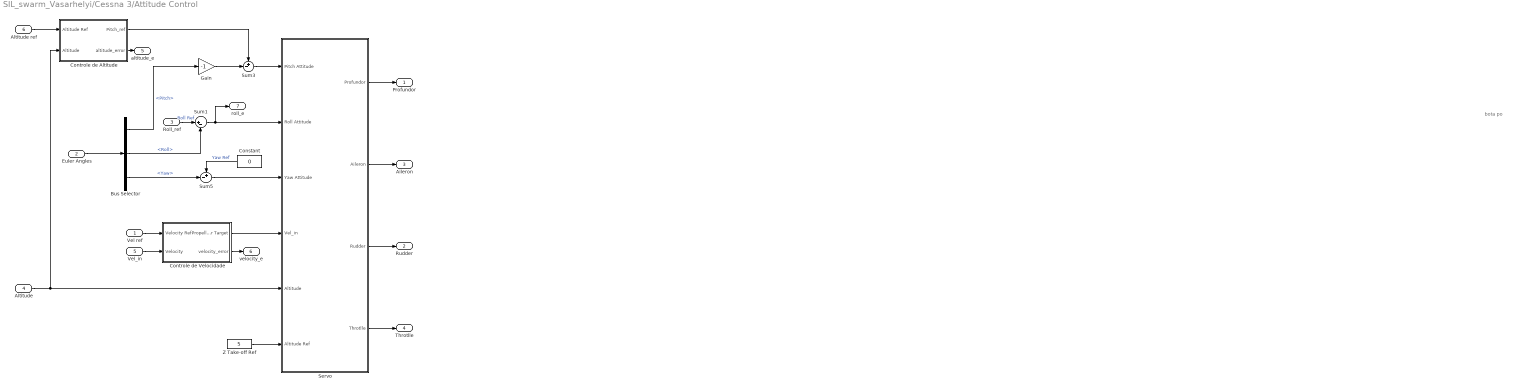
== system SIL_swarm_Vasarhelyi/Cessna 3/Attitude Control ==
  note: bota po
  Vel ref : Inport
  Euler Angles : Inport  Port=2
  Roll_ref : Inport  Port=3
  Altitude : Inport  Port=4
  Vel_in : Inport  Port=5
  Altitude ref : Inport  Port=6
  Bus Selector : BusSelector  OutputSignals=Pitch,Roll,Yaw
  Constant : Constant  Value=0
  Controle de Altitude : Subsystem
  Controle de Velocidade : Subsystem
  Gain : Gain  Gain=-1
  Servo : Subsystem
  Sum1 : Sum  Inputs=|+-
  Sum3 : Sum  Inputs=+-|
  Sum5 : Sum  Inputs=+-|
  Z Take-off Ref : Constant  Value=5
  Profundor : Outport
  Rudder : Outport  Port=2
  Aileron : Outport  Port=3
  Throtlle : Outport  Port=4
  altitude_e : Outport  Port=5
  velocity_e : Outport  Port=6
  roll_e : Outport  Port=7
  wires:
  Roll_ref/1 -> Sum1/1  "Roll Ref"
  Constant/1 -> Sum5/1  "Yaw Ref"
  Servo/4(Throtlle) -> Throtlle/1
  Servo/2(Aileron) -> Aileron/1
  Servo/3(Rudder) -> Rudder/1
  Servo/1(Profundor) -> Profundor/1
  Z Take-off Ref/1 -> Servo/6(Altitude Ref)
  Altitude/1 -> Controle de Altitude/2(Altitude), Servo/5(Altitude)
  Gain/1 -> Sum3/2
  Sum5/1 -> Servo/3(Yaw Attitude)
  Bus Selector/3 -> Sum5/2  "<Yaw>"
  Sum3/1 -> Servo/1(Pitch Attitude)
  Euler Angles/1 -> Bus Selector/1
  Bus Selector/1 -> Gain/1  "<Pitch>"
  Bus Selector/2 -> Sum1/2  "<Roll>"
  Controle de Velocidade/1(Propeller Target) -> Servo/4(Vel_in)
  Controle de Altitude/1(Pitch_ref) -> Sum3/1
  Vel ref/1 -> Controle de Velocidade/1(Velocity Ref)
  Altitude ref/1 -> Controle de Altitude/1(Altitude Ref)
  Sum1/1 -> roll_e/1, Servo/2(Roll Attitude)
  Vel_in/1 -> Controle de Velocidade/2(Velocity)
  Controle de Altitude/2(altitude_error) -> altitude_e/1
  Controle de Velocidade/2(velocity_error) -> velocity_e/1

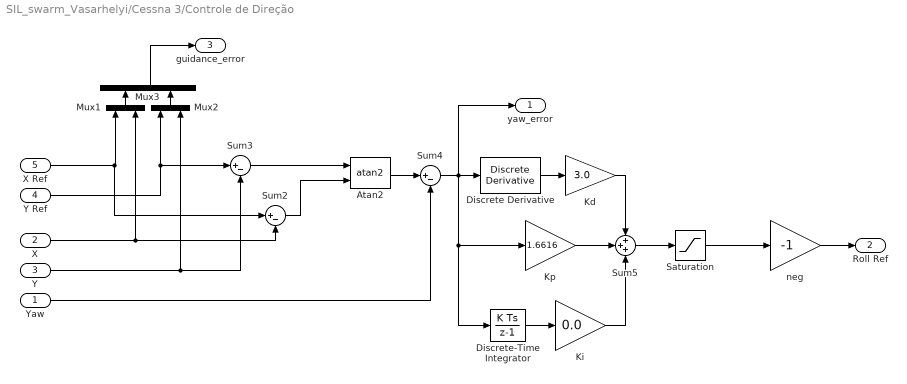
== system SIL_swarm_Vasarhelyi/Cessna 3/Controle de Direção ==
  Yaw : Inport
  X : Inport  Port=2
  Y : Inport  Port=3
  Y Ref : Inport  Port=4
  X Ref : Inport  Port=5
  Atan2 : Trigonometry  Operator=atan2
  Discrete Derivative : simulink/Discrete/Discrete Derivative  gainval=1.0  ICPrevScaledInput=0.0  OutMin=[]  OutMax=[]  OutDataType=fixdt(1, 16)  OutScaling=2^-10  DoSatur=off
  Discrete-Time Integrator : DiscreteIntegrator  SampleTime=-1  ICPrevOutput=DiscIntNeverNeededParam  ICPrevScaledInput=DiscIntNeverNeededParam
  Kd : Gain  Gain=3.0
  Ki : Gain  Gain=0.0
  Kp : Gain  Gain=1.6616
  Mux1 : Mux  Inputs=2
  Mux2 : Mux  Inputs=2
  Mux3 : Mux  Inputs=2
  Saturation : Saturate  UpperLimit=0.226893  LowerLimit=-0.226893
  Sum2 : Sum  Inputs=|+-
  Sum3 : Sum  Inputs=|+-
  Sum4 : Sum  Inputs=|+-
  Sum5 : Sum  Inputs=+++
  neg : Gain  Gain=-1
  yaw_error : Outport
  Roll Ref : Outport  Port=2
  guidance_error : Outport  Port=3
  wires:
  Mux1/1 -> Mux3/1
  Mux2/1 -> Mux3/2
  Saturation/1 -> neg/1
  neg/1 -> Roll Ref/1
  Sum3/1 -> Atan2/1
  Y/1 -> Sum3/2, Mux2/2
  Y Ref/1 -> Sum3/1, Mux2/1
  X Ref/1 -> Sum2/1, Mux1/1
  X/1 -> Sum2/2, Mux1/2
  Sum2/1 -> Atan2/2
  Atan2/1 -> Sum4/1
  Yaw/1 -> Sum4/2
  Mux3/1 -> guidance_error/1
  Sum5/1 -> Saturation/1
  Kp/1 -> Sum5/2
  Kd/1 -> Sum5/1
  Discrete Derivative/1 -> Kd/1
  Discrete-Time Integrator/1 -> Ki/1
  Sum4/1 -> Discrete-Time Integrator/1, Kp/1, Discrete Derivative/1, yaw_error/1
  Ki/1 -> Sum5/3

== system SIL_swarm_Vasarhelyi/Cessna 3/High-Level ==
  Pos : Inport
  Altitude ref : Inport  Port=2
  Xi : Inport  Port=3
  Bus Selector2 : BusSelector  OutputSignals=X,Y,Altitude
  Filtered Derivative Discrete : eeGeneralControl/Filtered Derivative (Discrete or Continuous)  K=1  T=0.001  B=inf  A=-inf  minRatio=10  init_option=Inherited from block input  x0=0  Ts=-1
      settings: SourceProductBaseCode=PS
  Gerador de Waypoints : Subsystem
  Mux : Mux  Inputs=3
  Mux1 : Mux  Inputs=3
  Terminator2 : Terminator
  Vasarhelyi Algorithm : Subsystem
  Velocity Direction : MATLAB Function  TreatAsAtomicUnit=on
  Y Ref : Outport
  X Ref : Outport  Port=2
  vel : Outport  Port=3
  u_ref : Outport  Port=4
  Waypoints : Outport  Port=5
  wires:
  Mux1/1 -> Waypoints/1, Velocity Direction/2(wp)
  Velocity Direction/1(u_ref) -> u_ref/1, Vasarhelyi Algorithm/3(u_ref)
  Pos/1 -> Bus Selector2/1
  Altitude ref/1 -> Mux1/3
  Gerador de Waypoints/2(Y Ref) -> Mux1/2
  Gerador de Waypoints/1(X Ref) -> Mux1/1
  Bus Selector2/1 -> Mux/1  "<X>"
  Bus Selector2/2 -> Mux/2  "<Y>"
  Bus Selector2/3 -> Mux/3  "<Altitude>"
  Mux/1 -> Filtered Derivative Discrete/1, Vasarhelyi Algorithm/1(pos_i), Velocity Direction/1(pos)
  Filtered Derivative Discrete/1 -> vel/1
  Xi/1 -> Vasarhelyi Algorithm/2(pqj)
  Vasarhelyi Algorithm/1(X) -> X Ref/1
  Vasarhelyi Algorithm/2(Y) -> Y Ref/1
  Vasarhelyi Algorithm/3(Z) -> Terminator2/1
  Vasarhelyi Algorithm/4(Xi) -> Gerador de Waypoints/1(Xi)

== system SIL_swarm_Vasarhelyi/Cessna 3/ROS Communication ==
  Profundor : Inport
  Rudder : Inport  Port=2
  Aileron : Inport  Port=3
  Throttle : Inport  Port=4
  Constant : Constant  Value=0
  Constant1 : Constant  Value=0
  Envio e Recepção de Dados do ROS : Subsystem
  Terminator2 : Terminator
  Roll : Outport
  Pitch : Outport  Port=2
  Yaw : Outport  Port=3
  ECEF Y : Outport  Port=4
  ECEF X : Outport  Port=5
  ECEF Z : Outport  Port=6
  Velocity : Outport  Port=7
  Xi : Outport  Port=8
  wires:
  Profundor/1 -> Envio e Recepção de Dados do ROS/2(Elevators)
  Constant/1 -> Envio e Recepção de Dados do ROS/3(Flap)
  Aileron/1 -> Envio e Recepção de Dados do ROS/4(Aileron)
  Envio e Recepção de Dados do ROS/1(Pitch) -> Pitch/1
  Envio e Recepção de Dados do ROS/4(ECEF X) -> ECEF X/1
  Envio e Recepção de Dados do ROS/5(ECEF Y) -> ECEF Y/1
  Envio e Recepção de Dados do ROS/2(Yaw) -> Yaw/1
  Envio e Recepção de Dados do ROS/3(Roll) -> Roll/1
  Envio e Recepção de Dados do ROS/6(ECEF Z) -> ECEF Z/1
  Envio e Recepção de Dados do ROS/7(Velocity) -> Velocity/1
  Rudder/1 -> Terminator2/1
  Envio e Recepção de Dados do ROS/8(Xi) -> Xi/1
  Throttle/1 -> Envio e Recepção de Dados do ROS/5(Propeller)
  Constant1/1 -> Envio e Recepção de Dados do ROS/1(Rudder)

== system SIL_swarm_Vasarhelyi/Cessna 4/Attitude Control ==
  note: bota po
  Vel ref : Inport
  Euler Angles : Inport  Port=2
  Roll_ref : Inport  Port=3
  Altitude : Inport  Port=4
  Vel_in : Inport  Port=5
  Altitude ref : Inport  Port=6
  Bus Selector : BusSelector  OutputSignals=Pitch,Roll,Yaw
  Constant : Constant  Value=0
  Controle de Altitude : Subsystem
  Controle de Velocidade : Subsystem
  Gain : Gain  Gain=-1
  Servo : Subsystem
  Sum1 : Sum  Inputs=|+-
  Sum3 : Sum  Inputs=+-|
  Sum5 : Sum  Inputs=+-|
  Z Take-off Ref : Constant  Value=5
  Profundor : Outport
  Rudder : Outport  Port=2
  Aileron : Outport  Port=3
  Throtlle : Outport  Port=4
  altitude_e : Outport  Port=5
  velocity_e : Outport  Port=6
  roll_e : Outport  Port=7
  wires:
  Roll_ref/1 -> Sum1/1  "Roll Ref"
  Constant/1 -> Sum5/1  "Yaw Ref"
  Servo/4(Throtlle) -> Throtlle/1
  Servo/2(Aileron) -> Aileron/1
  Servo/3(Rudder) -> Rudder/1
  Servo/1(Profundor) -> Profundor/1
  Z Take-off Ref/1 -> Servo/6(Altitude Ref)
  Altitude/1 -> Controle de Altitude/2(Altitude), Servo/5(Altitude)
  Gain/1 -> Sum3/2
  Sum5/1 -> Servo/3(Yaw Attitude)
  Bus Selector/3 -> Sum5/2  "<Yaw>"
  Sum3/1 -> Servo/1(Pitch Attitude)
  Euler Angles/1 -> Bus Selector/1
  Bus Selector/1 -> Gain/1  "<Pitch>"
  Bus Selector/2 -> Sum1/2  "<Roll>"
  Controle de Velocidade/1(Propeller Target) -> Servo/4(Vel_in)
  Controle de Altitude/1(Pitch_ref) -> Sum3/1
  Vel ref/1 -> Controle de Velocidade/1(Velocity Ref)
  Altitude ref/1 -> Controle de Altitude/1(Altitude Ref)
  Sum1/1 -> roll_e/1, Servo/2(Roll Attitude)
  Vel_in/1 -> Controle de Velocidade/2(Velocity)
  Controle de Altitude/2(altitude_error) -> altitude_e/1
  Controle de Velocidade/2(velocity_error) -> velocity_e/1
